simulink model "cartesian_impedance_control"  (R2022b)
settings: Solver=FixedStepDiscrete  StartTime=0.0  StopTime=inf  FixedStep=0.001  RelTol=1e-3
PreLoadFcn:
  | set_param(gcs, 'RTWSystemTargetFile', 'franka_emika_panda.tlc');
  | 
  | demos_common_configs();
  | collision_behavior = ones(1,52)*100;
InitFcn:
  | parameters;
values from neighbouring files (symbols this model uses):
  init_guess_0 = [2.22044604925e-16 2.22044604925e-16 2.22044604925e-16 2.22044604925e-16 2.22044604925e-16 2.22044604925e-16 2.22044604925e-16 2.22044604925e-16 2.22044604925e-16 2.22044604925e-16 2.22044604925e-16 2.22044604925e-16 ... (276 elements, 276x1)]    [mpc_init_guess_test.mat]    (also in parameters.m = param_MPC8_init_guess.init_guess(2,:))
  mpc_init_reference_values = [-0.0348999931742 -2.4612999645 -3.55689998059 2.23979998651 0.0349999704327 -1.24879998892 0 0 0 0 0 0 ... (54 elements, 54x1)]    [mpc_init_ref_test.mat]
  param_weight_init_cell = [100 0 0 0 0 0 0 100 0 0 0 0 ... (180 elements, 1x180)]    [mpc_init_weight_test.mat]
  q_init = [0, -pi/4, 0, -3 * pi/4, 0, pi/2, pi/4]'    [parameters.m]    (also in parameters_franka_fr3.m)
undefined symbols (not defined in the file or in its folder): ctrl_param, param_robot
libraries: franka_simulink_library x5, dspnetwork x2
settings Model: SimulationMode=external  ExtModeTrigDuration=10000  Creator=vasi_ko  LastModifiedBy=rslstudent
settings SolverCC: AlgebraicLoopSolver=TrustRegion
settings DataIOCC: LimitDataPoints=on  SaveFormat=Array  ReturnWorkspaceOutputs=off
settings OptimizationCC: EnhancedBackFolding=on  OptimizeBlockOrder=speed  DifferentSizesBufferReuse=on  OptimizationCustomize=off
settings DebuggingCC: SolverPrmCheckMsg=warning  ParameterTunabilityLossMsg=error  UnconnectedInputMsg=warning  UnconnectedOutputMsg=warning  UnconnectedLineMsg=warning  SFUnexpectedBacktrackingDiag=warning  SFNoUnconditionalDefaultTransitionDiag=warning  SFExecutionAtInitializationDiag=none  SFMachineParentedDataDiag=warning  ArithmeticOperatorsInVariantConditions=warning
settings HardwareCC: ProdBitPerLong=64  ProdHWDeviceType=Intel->x86-64 (Linux 64)
settings ModelReferenceCC: EnableRefExpFcnMdlSchedulingChecks=on  PropagateSignalLabelsOutOfModel=off
settings SFSimCC: SimUseLocalCustomCode=off  MATLABDynamicMemAlloc=off  CustomCodeUndefinedFunction=UseInterfaceOnly  SimTargetLang=C++
settings RTWCC: SystemTargetFile=franka_emika_panda.tlc  RTWUseLocalCustomCode=off  Toolchain=Franka Simulink | gmake (64-bit linux)  BuildConfiguration=Faster Runs  TargetLang=C++
settings CodeAppCC: OperatorAnnotations=on
settings STFCustomTargetCC: TargetLangStandard=C99 (ISO)  ModelReferenceCompliant=off  MatFileLogging=on  GRTInterface=on  UseToolchainInfoCompliant=on  SystemTargetFile=franka_emika_panda.tlc
settings GRTTargetCC: ModelReferenceCompliant=off  ParMdlRefBuildCompliant=off  CompOptLevelCompliant=off  ConcurrentExecutionCompliant=off  CombineOutputUpdateFcns=off  CPPClassGenCompliant=off  GRTInterface=on  ExtModeStaticAlloc=on  ExtModeTransport=1  ExtModeMexFile=ext_xcp  ExtModeIntrfLevel=Level2 - Open
settings ConfigComp: CovMetricSettings=dw  CovSaveCumulativeToWorkspaceVar=on  CovSaveSingleToWorkspaceVar=on  CovExternalEMLEnable=off  CovSFcnEnable=off

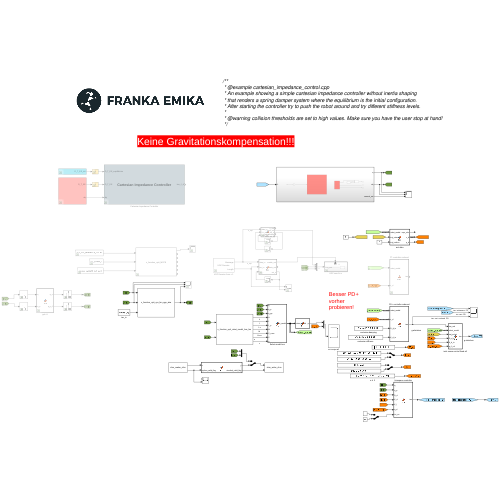
[thumbnail: Simulink's stored preview of the top-level diagram]
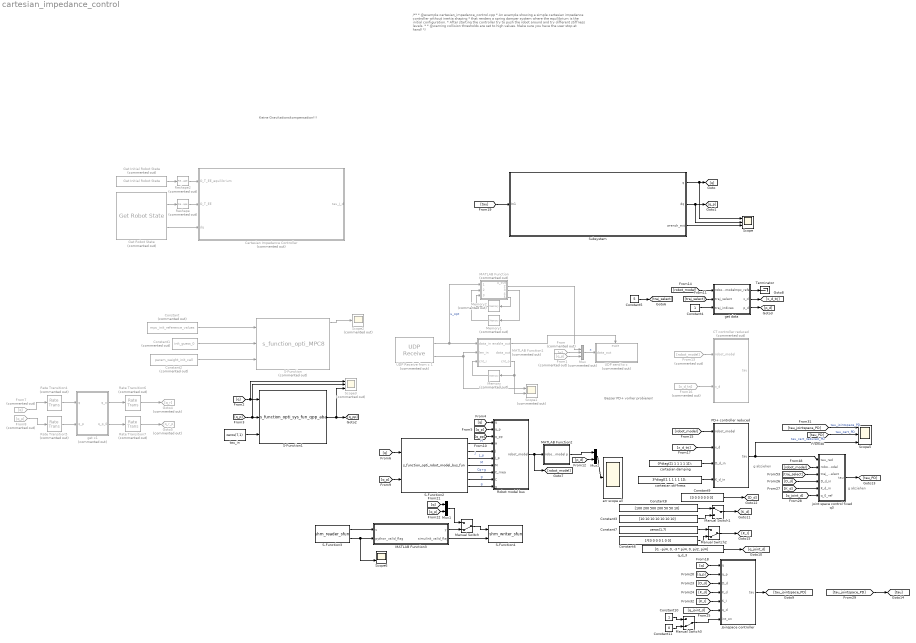
== system cartesian_impedance_control ==
  note: g abziehen
  note: Keine Gravitationskompensation!!!
  note: /**
      |  * @example cartesian_impedance_control.cpp
      |  * An example showing a simple cartesian impedance controller without inertia shaping
      |  * that renders a spring damper system where the equilibrium is the initial configuration.
      |  * After starting the controller try to push the robot around and try different stiffness levels.
      |  *
      |  * @warning collision thresholds are set to high values. Make sure you have the user stop at hand!
      |  */
  note: Besser PD+ vorher probieren!
  note: g abziehen
  CT controller reduced : MATLAB Function  Commented=on  TreatAsAtomicUnit=on
  Cartesian Impedance Controller : Subsystem  Commented=on
      mask Display:
      | disp('{\bf\fontsize{18}Cartesian Impedance Controller}', 'texmode','on');
      | 
      | block_icon('Controller')
      | 
      | port_label('output',1,'tau_J_d');
      | 
      | port_label('input',1,'O_T_EE_equilibrium');
      | port_label('input',2,'O_T_EE');
      | port_label('input',3,'dq');
  Constant : Constant  Commented=on  Value=mpc_init_reference_values
  Constant1 : Constant  Commented=on  Value=init_guess_0
  Constant10 : Constant
  Constant11 : Constant  Value=0
  Constant2 : Constant  Commented=on  Value=param_weight_init_cell
  Constant3 : Constant  Value=[10 10 10 10 10 10 10]
  Constant4 : Constant
  Constant5 : Constant  Value=5
  Constant6 : Constant  Value=1*[0 0 0 0 1 0 0]
  Constant7 : Constant  Value=zeros(1,7)
  Constant8 : Constant  Value=[100 200 500 200 50 50 10]
  Constant9 : Constant  Value=[0 0 0 0 0 0 0]
  From : From  Commented=on  GotoTag=q
  From1 : From  Commented=on  GotoTag=q_p
  From13 : From  Commented=on  GotoTag=robot_model
  From16 : From  Commented=on  GotoTag=x_d_trj
  From7 : From  Commented=on  GotoTag=q
  From8 : From  Commented=on  GotoTag=q_p
  Get Initial Robot State : franka_simulink_library/Get Initial Robot State  Commented=on  robot_ip=robot_ip  signals_requested='O_T_EE'
      settings: SourceProductName=Franka Emika Simulink Support Package
  Get Robot State : franka_simulink_library/Get Robot State  Commented=on  robot_ip=robot_ip  signals_requested='O_T_EE dq'
      settings: SourceProductName=Franka Emika Simulink Support Package
  Goto4 : Goto  Commented=on  GotoTag=q_r
  Goto5 : Goto  Commented=on  GotoTag=q_r_p
  Joinspace controller : MATLAB Function  TreatAsAtomicUnit=on
  MATLAB Function : MATLAB Function  Commented=on  TreatAsAtomicUnit=on
  MATLAB Function1 : MATLAB Function  Commented=on  TreatAsAtomicUnit=on
  MATLAB Function2 : MATLAB Function  TreatAsAtomicUnit=on
  MATLAB Function3 : MATLAB Function  TreatAsAtomicUnit=on
  Manual Switch : ManualSwitch  CurrentSetting=0
  Manual Switch1 : ManualSwitch
  Manual Switch2 : ManualSwitch  CurrentSetting=0
  Manual Switch3 : ManualSwitch  CurrentSetting=0
  Memory : Memory  Commented=on
  Memory1 : Memory  Commented=on
  Memory2 : Memory  Commented=on
  Mux : Mux  Commented=on  Inputs=3
  Mux1 : Mux  Inputs=2
  Mux2 : Mux  Inputs=2
  PD+ controller reduced : MATLAB Function  TreatAsAtomicUnit=on
  Rate Transition4 : RateTransition  Commented=on  OutPortSampleTime=1e-2
  Rate Transition5 : RateTransition  Commented=on  OutPortSampleTime=1e-2
  Rate Transition6 : RateTransition  Commented=on
  Rate Transition7 : RateTransition  Commented=on
  Reshape : Reshape  Commented=on  OutputDimensionality=Customize  OutputDimensions=[4,4]
  Reshape2 : Reshape  Commented=on  OutputDimensionality=Customize  OutputDimensions=[4,4]
  Robot model bus : MATLAB Function  TreatAsAtomicUnit=on
  S-Function : S-Function  Commented=on  FunctionName=s_function_opti_MPC8  SFunctionModules='MPC8'  SFunctionDeploymentMode=off  EnableBusSupport=off
  S-Function1 : S-Function  FunctionName=s_function_opti_sys_fun_qpp_aba  SFunctionModules='sys_fun_qpp_aba'  SFunctionDeploymentMode=off  EnableBusSupport=off
  S-Function2 : S-Function  FunctionName=s_function_opti_robot_model_bus_fun  SFunctionModules='robot_model_bus_fun'  SFunctionDeploymentMode=off  EnableBusSupport=off
  S-Function3 : S-Function  FunctionName=shm_reader_sfun  Parameters='data_from_python', 'data_from_python_valid'  SFunctionDeploymentMode=off  EnableBusSupport=off
  S-Function4 : S-Function  FunctionName=shm_writer_sfun  Parameters='data_from_simulink', 'data_from_simulink_valid'  SFunctionDeploymentMode=off  EnableBusSupport=off
  Scope : Scope  NumInputPorts=3
  Scope1 : Scope  Commented=on  NumInputPorts=2
  Scope2 : Scope  Commented=on
  Scope3 : Scope  Commented=on  NumInputPorts=3
  Scope5 : Scope  NumInputPorts=3
  Scope6 : Scope  NumInputPorts=2
  Subsystem : Subsystem
  Terminator : Terminator
  UDP Receive from c 1 : dspnetwork/UDP Receive  Commented=on  localURL='0.0.0.0'  localPort=8080  remoteURL='127.0.0.1'  remotePort=-1  recvBufferSize=8+6*8*5  dims=1+6*5  signalDatatype=double  isComplex=off  isVarSize=off  showBlockingTime=off  blockingTime=0  sampletime=param_global.Ta  blockPlatform=[]
      settings: LibrarySourceBlock=dspsrcs4/UDP Receive
  UDP send to c : Subsystem  Commented=on
  cartesian damping : Constant  Value=0*diag([1 1 1 1 1 1]);
  cartesian stiffness : Constant  Value=3*diag([1 1 1 1 1 1]);
  err scope all : Scope
  get data : MATLAB Function  TreatAsAtomicUnit=on
  get x1 : MATLAB Function  Commented=on  TreatAsAtomicUnit=on
  joint space control fixed q3 : MATLAB Function  TreatAsAtomicUnit=on
  q_d_3 : Constant  Value=[0, -pi/4, 0, -3 * pi/4, 0, pi/2, pi/4]
  tau_in : Constant  Value=zeros(7,1)
  wires:
  Reshape2/1 -> Cartesian Impedance Controller/1(O_T_EE_equilibrium)
  get data/1(mpc_refs) -> Terminator/1
  From16/1 -> CT controller reduced/2(x_d)
  MATLAB Function/3(init_cnt_o) -> Memory1/1
  MATLAB Function/2(send_cnt) -> Mux/1
  [robot_model] -> get data/1(robot_model)
  MATLAB Function1/3(cnt_o) -> Scope1/2, Memory/1
  Get Initial Robot State/1 -> Reshape2/1
  tau_in/1 -> S-Function1/3
  S-Function2/3 -> Robot model bus/6(J_p)  "J_p"
  [x_d_trj] -> PD+ controller reduced/2(x_d)
  Memory1/1 -> MATLAB Function/2(init_cnt)
  Rate Transition7/1 -> Goto5/1
  [q_p] -> Scope3/2, S-Function1/2
  From/1 -> Mux/2
  Subsystem/1(q) -> Scope/1, [q]
  Constant2/1 -> S-Function/3
  Subsystem/2(dq) -> Scope/2, [q_p]
  [robot_model] -> PD+ controller reduced/1(robot_model)
  S-Function2/6 -> Robot model bus/9(C)  "g"
  [q_pp] -> Robot model bus/3(q_pp)
  [q] -> Scope3/1, S-Function1/1
  UDP Receive from c 1/1 -> MATLAB Function/1(data_in), MATLAB Function1/1(data_in)  "u_opt"
  Constant1/1 -> S-Function/2
  Get Robot State/2 -> Cartesian Impedance Controller/3(dq)
  Rate Transition5/1 -> get x1/2(q_p)
  UDP Receive from c 1/2 -> MATLAB Function1/2(len_in), Scope1/1
  MATLAB Function/5(data_cnt_o) -> Memory2/1
  get x1/1(q_o) -> Rate Transition6/1
  From8/1 -> Rate Transition5/1
  From7/1 -> Rate Transition4/1
  get data/2(x_d) -> [x_d_trj]
  S-Function2/5 -> Robot model bus/8(C_rnea)  "Cq+g"
  S-Function1/1 -> [q_pp], Scope3/3
  Rate Transition6/1 -> Goto4/1
  S-Function2/1 -> Robot model bus/4(H)  "H"
  Reshape/1 -> Cartesian Impedance Controller/2(O_T_EE)
  get x1/2(q_p_0) -> Rate Transition7/1
  MATLAB Function1/1(enable_out) -> UDP send to c/Enable
  Mux/1 -> UDP send to c/1(data_out)  "x"
  S-Function2/2 -> Robot model bus/5(J)  "J"
  Get Robot State/1 -> Reshape/1
  S-Function2/4 -> Robot model bus/7(M)  "M"
  Robot model bus/1(robot_model) -> MATLAB Function2/1(robot_model), [robot_model]
  Subsystem/3(wrench_ext) -> Scope/3
  S-Function/1 -> Scope2/1
  Memory/1 -> MATLAB Function1/3(cnt_i)
  Memory2/1 -> MATLAB Function/3(data_cnt)
  From1/1 -> Mux/3
  Constant/1 -> S-Function/1
  From13/1 -> CT controller reduced/1(robot_model)
  S-Function2/7 -> Robot model bus/10(g)  "g"
  Rate Transition4/1 -> get x1/1(q)
  Constant4/1 -> get data/3(traj_indices)
  cartesian stiffness/1 -> PD+ controller reduced/4(K_d_in)
  cartesian damping/1 -> PD+ controller reduced/3(D_d_in)
  Joinspace controller/1(tau) -> [tau_jointspace_PD]
  [tau] -> Subsystem/1(In1)
  [q] -> Joinspace controller/1(q)
  [q_p] -> Joinspace controller/2(q_p)
  S-Function3/1 -> MATLAB Function3/1(u)
  S-Function3/2 -> Scope6/2, MATLAB Function3/2(python_valid_flag)
  MATLAB Function3/2(simulink_valid_flag) -> S-Function4/2
  [q] -> Mux1/1
  [q_p] -> Mux1/2
  MATLAB Function3/1(y) -> Manual Switch/2
  Manual Switch/1 -> S-Function4/1
  Mux1/1 -> Manual Switch/1
  [q] -> Robot model bus/1(q)
  [q_p] -> Robot model bus/2(q_p)
  [q] -> S-Function2/1
  [q_p] -> S-Function2/2
  get data/3(p_d) -> [p_d]
  [p_d] -> Mux2/2
  MATLAB Function2/1(p) -> Mux2/1
  Mux2/1 -> err scope all/1
  [robot_model] -> joint space control fixed q3/2(robot_model)
  PD+ controller reduced/1(tau) -> Scope5/3, joint space control fixed q3/1(tau_red)  "tau_cart_reduced_PD"
  [traj_select] -> joint space control fixed q3/3(traj_select)
  [traj_select] -> get data/2(traj_select)
  Constant5/1 -> [traj_select]
  [q_joint_d] -> Joinspace controller/6(q_d)
  q_d_3/1 -> [q_joint_d]
  [K_d] -> Joinspace controller/4(K_d)
  [D_d] -> Joinspace controller/3(D_d)
  Constant9/1 -> [D_d]
  [D_d] -> joint space control fixed q3/4(D_d_in)
  [K_d] -> joint space control fixed q3/5(K_d_in)
  [q_joint_d] -> joint space control fixed q3/6(q_0_ref)
  joint space control fixed q3/1(tau) -> [tau_PD]
  [tau_jointspace_PD] -> [tau]
  [tau_PD] -> Scope5/2  "tau_cart_PD"
  [tau_jointspace_PD] -> Scope5/1  "tau_jointspace_PD"
  Constant8/1 -> Manual Switch1/1
  Constant3/1 -> Manual Switch1/2
  Manual Switch1/1 -> [K_d]
  [K_I] -> Joinspace controller/5(K_I)
  Manual Switch2/1 -> [K_I]
  Constant6/1 -> Manual Switch2/2
  Constant7/1 -> Manual Switch2/1
  Constant10/1 -> Manual Switch3/1
  Constant11/1 -> Manual Switch3/2
  Manual Switch3/1 -> Joinspace controller/7(int_on)

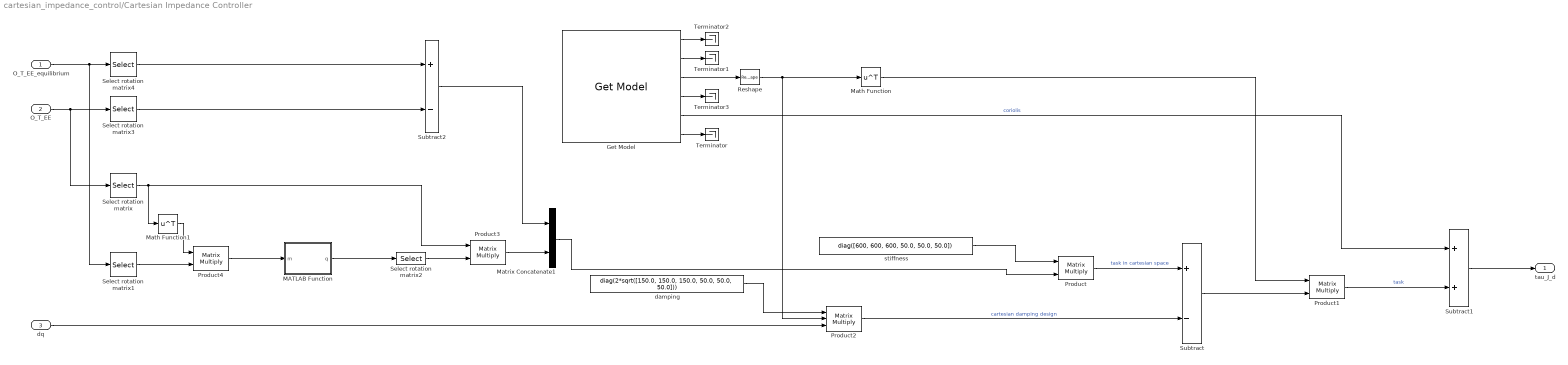
== system cartesian_impedance_control/Cartesian Impedance Controller ==
  O_T_EE_equilibrium : Inport
  O_T_EE : Inport  Port=2
  dq : Inport  Port=3
  Get Model : franka_simulink_library/Get Model  robot_ip=robot_ip
      settings: SourceProductName=Franka Emika Simulink Support Package
  MATLAB Function : MATLAB Function  TreatAsAtomicUnit=on
  Math Function : Math  Operator=transpose  SignedPower=on
  Math Function1 : Math  Operator=transpose  SignedPower=on
  Matrix Concatenate1 : Concatenate
  Product{,1,3..4} (4 alike) : Product  Multiplication=Matrix(*)
  Product2 : Product  Inputs=3  Multiplication=Matrix(*)
  Reshape : Reshape  OutputDimensionality=Customize  OutputDimensions=[6,7]
  Select rotation matrix : Selector  NumberOfDimensions=2  InputPortWidth=3  IndexOptions=Index vector (dialog),Index vector (dialog)  Indices=[1,2,3],[1 2 3]  OutputSizes=1
  Select rotation matrix1 : Selector  NumberOfDimensions=2  InputPortWidth=3  IndexOptions=Index vector (dialog),Index vector (dialog)  Indices=[1,2,3],[1 2 3]  OutputSizes=1
  Select rotation matrix2 : Selector  InputPortWidth=4  IndexOptions=Index vector (dialog)  Indices=[2,3,4]  OutputSizes=1
  Select rotation matrix3 : Selector  NumberOfDimensions=2  InputPortWidth=3  IndexOptions=Index vector (dialog),Index vector (dialog)  Indices=[1,2,3],[4]  OutputSizes=1
  Select rotation matrix4 : Selector  NumberOfDimensions=2  InputPortWidth=3  IndexOptions=Index vector (dialog),Index vector (dialog)  Indices=[1,2,3],[4]  OutputSizes=1
  Subtract : Sum  Inputs=+-
  Subtract1 : Sum
  Subtract2 : Sum  Inputs=+-
  Terminator{,1..3} (4 alike) : Terminator
  damping : Constant  Value=diag(2*sqrt([150.0, 150.0, 150.0, 50.0, 50.0, 50.0]))  VectorParams1D=off
  stiffness : Constant  Value=diag([600, 600, 600, 50.0, 50.0, 50.0])  VectorParams1D=off
  tau_J_d : Outport  VectorParamsAs1DForOutWhenUnconnected=off
  wires:
  Get Model/6 -> Terminator/1
  Get Model/2 -> Terminator1/1
  Get Model/1 -> Terminator2/1
  Get Model/4 -> Terminator3/1
  Get Model/3 -> Reshape/1
  Reshape/1 -> Product2/2, Math Function/1
  stiffness/1 -> Product/1
  Math Function/1 -> Product1/1
  Product/1 -> Subtract/1  "task in cartesian space"
  Product2/1 -> Subtract/2  "cartesian damping design"
  Get Model/5 -> Subtract1/1  "coriolis"
  dq/1 -> Product2/3
  damping/1 -> Product2/1
  Subtract1/1 -> tau_J_d/1
  Product1/1 -> Subtract1/2  "task"
  O_T_EE/1 -> Select rotation matrix3/1, Select rotation matrix/1
  O_T_EE_equilibrium/1 -> Select rotation matrix4/1, Select rotation matrix1/1
  Select rotation matrix4/1 -> Subtract2/1
  Select rotation matrix3/1 -> Subtract2/2
  Subtract2/1 -> Matrix Concatenate1/1
  MATLAB Function/1(q) -> Select rotation matrix2/1
  Product4/1 -> MATLAB Function/1(m)
  Subtract/1 -> Product1/2
  Select rotation matrix2/1 -> Product3/2
  Matrix Concatenate1/1 -> Product/2
  Select rotation matrix/1 -> Math Function1/1, Product3/1
  Product3/1 -> Matrix Concatenate1/2
  Select rotation matrix1/1 -> Product4/2
  Math Function1/1 -> Product4/1

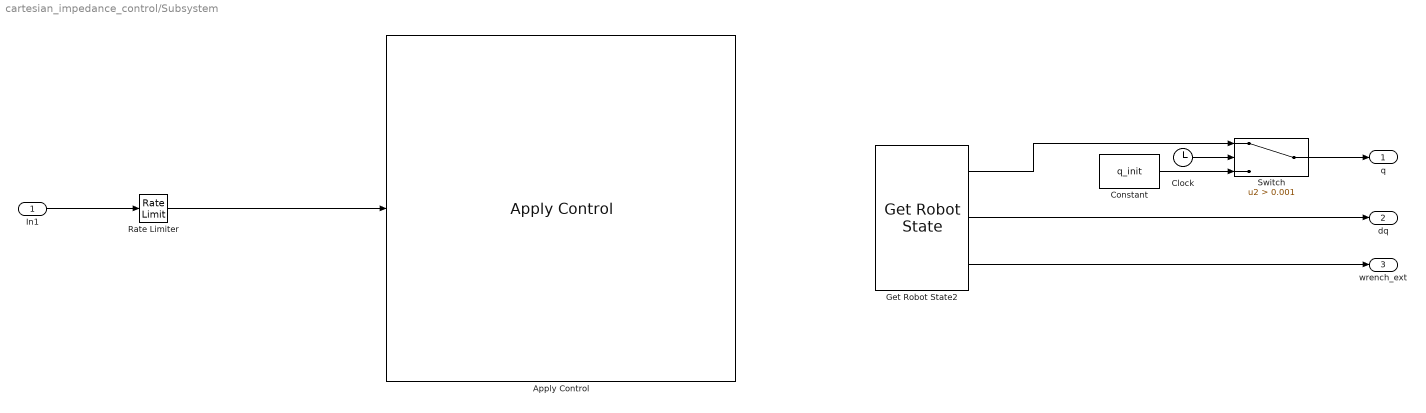
== system cartesian_impedance_control/Subsystem ==
  In1 : Inport
  Apply Control : franka_simulink_library/Apply Control  robot_ip=robot_ip  gripper_attached=off  control_mode=Torque Control  controller_choice=Joint Impedance Controller  elbow_control=on  collision_thresholds=100*ones(1,52)  joint_impedance=joint_impedance  cartesian_impedance=cartesian_impedance  load_inertia=load_inertia  EE_T_K=EE_T_K  init_joint_configuration_req=on  init_joint_configuration=q_init'
      settings: SourceProductName=Franka Emika Simulink Support Package
  Clock : Clock
  Constant : Constant  Value=q_init
  Get Robot State2 : franka_simulink_library/Get Robot State  robot_ip=robot_ip  signals_requested='q dq O_F_ext_hat_K'
      settings: SourceProductName=Franka Emika Simulink Support Package
  Rate Limiter : RateLimiter  RisingSlewLimit=1000  FallingSlewLimit=-1000  SampleTimeMode=inherited
  Switch : Switch  Criteria=u2 > Threshold  Threshold=0.001  SaturateOnIntegerOverflow=off  InputSameDT=off
  q : Outport
  dq : Outport  Port=2
  wrench_ext : Outport  Port=3
  wires:
  Clock/1 -> Switch/2
  Constant/1 -> Switch/3
  Get Robot State2/3 -> wrench_ext/1
  Get Robot State2/2 -> dq/1
  In1/1 -> Rate Limiter/1
  Get Robot State2/1 -> Switch/1
  Switch/1 -> q/1
  Rate Limiter/1 -> Apply Control/1

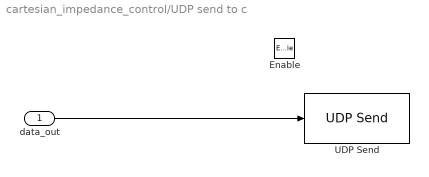
== system cartesian_impedance_control/UDP send to c ==
  data_out : Inport
  Enable : EnablePort
  UDP Send : dspnetwork/UDP Send  remoteURL='127.0.0.1'  remotePort=8081  localURL='0.0.0.0'  localPortSource=Automatically determine  localPort=8081  sendBufferSize=104  sampletime=-1  blockPlatform=[]  separateLengthPort=0
      settings: LibrarySourceBlock=dspsnks4/UDP Send
  wires:
  data_out/1 -> UDP Send/1

== matlab function cartesian_impedance_control/get data ==
  settings: updateMethod=DISCRETE  sampleTime=param_global.Ta
  data: mpc_refs output; robot_model input Bus: robot_model; traj_select input; param_traj_data parameter; traj_indices input; x_d output Bus: x_d; p_d output
function [mpc_refs, x_d, p_d]  = fcn(robot_model, traj_select, param_traj_data, traj_indices)
persistent cnt;

if(isempty(cnt))
    cnt = 1;
end

traj_indices = traj_indices + (cnt-1);

% Parameters
q    = robot_model.q;      % generalized coordinates
q_p  = robot_model.q_p;  % time derivative of generalized coordinates

x_k = [q;q_p];

% Assemble vector of recieved output measurements
p_d     = param_traj_data.p_d(   1:3, traj_indices, traj_select);
q_d     = param_traj_data.q_d(   1:4, traj_indices, traj_select);

y_d = [p_d; q_d];

%% Reference out
mpc_refs = [x_k(:); y_d(:)];

%% Offline Trajectory out
x_d.p_d            = param_traj_data.p_d(           :,    cnt, traj_select);
x_d.p_d_p          = param_traj_data.p_d_p(         :,    cnt, traj_select);
x_d.p_d_pp         = param_traj_data.p_d_pp(        :,    cnt, traj_select);
x_d.Phi_d          = param_traj_data.Phi_d(         :,    cnt, traj_select);
x_d.Phi_d_p        = param_traj_data.Phi_d_p(       :,    cnt, traj_select);
x_d.Phi_d_pp       = param_traj_data.Phi_d_pp(      :,    cnt, traj_select);
x_d.R_d            = param_traj_data.R_d(           :, :, cnt, traj_select);
x_d.q_d            = param_traj_data.q_d(           :,    cnt, traj_select);
x_d.q_d_p          = param_traj_data.q_d_p(         :,    cnt, traj_select);
x_d.q_d_pp         = param_traj_data.q_d_pp(        :,    cnt, traj_select);
x_d.omega_d        = param_traj_data.omega_d(       :,    cnt, traj_select);
x_d.omega_d_p      = param_traj_data.omega_d_p(     :,    cnt, traj_select);
x_d.alpha_d        = param_traj_data.alpha_d(       :,    cnt, traj_select);
x_d.alpha_d_p      = param_traj_data.alpha_d_p(     :,    cnt, traj_select);
x_d.alpha_d_pp     = param_traj_data.alpha_d_pp(    :,    cnt, traj_select);
x_d.rot_ax_d       = param_traj_data.rot_ax_d(      :,    cnt, traj_select);
x_d.alpha_d_offset = param_traj_data.alpha_d_offset(:,    cnt, traj_select);
x_d.q_d_rel        = param_traj_data.q_d_rel(       :,    cnt, traj_select);

%if(cnt < param_traj_data.N)
    %cnt = cnt+1;
%end

== matlab function cartesian_impedance_control/Joinspace controller ==
  settings: updateMethod=DISCRETE  sampleTime=param_global.Ta
  data: tau output; q input; q_p input; D_d input; K_d input; K_I input; q_d input; int_on input
function tau  = fcn(q, q_p, D_d, K_d, K_I, q_d, int_on)

% Parameters
persistent e_I;
if(isempty(e_I))
    e_I = zeros(7,1);
end

e_q = q - q_d;
tau = -diag(D_d)*q_p -diag(K_d)*e_q;

if(int_on == 1)
    e_I = e_I + e_q;
    tau_I = -diag(K_I) * e_I;
else
    e_I = zeros(7,1);
    tau_I = zeros(7,1);
end
tau = tau + tau_I;

== matlab function cartesian_impedance_control/MATLAB Function3 ==
  settings: updateMethod=DISCRETE  sampleTime=1e-3
  data: u input; y output; simulink_valid_flag output; python_valid_flag input
function [y, simulink_valid_flag] = fcn(u, python_valid_flag)

if(python_valid_flag == 1)
    y = u(1:14);
    simulink_valid_flag = 1;
else
    y = zeros(14,1);
    simulink_valid_flag = 0;
end

== matlab function cartesian_impedance_control/CT controller reduced ==
  settings: updateMethod=DISCRETE  sampleTime=param_global.Ta
  data: tau output; robot_model input Bus: robot_model; x_d input Bus: x_d; ctrl_param parameter; param_robot parameter
function tau  = fcn(robot_model, x_d, ctrl_param, param_robot)

% Parameters
%q = robot_model.q;      % generalized coordinates
q_p = robot_model.q_p;  % time derivative of generalized coordinates

M = robot_model.M;      % inertia matrix
%C = robot_model.C;      % coriolis matrix
%g = robot_model.g;      % gravitational forces
%C_rnea = C*q_p + g;
C_rnea = robot_model.C_rnea; % C_rnea(q, q_p) = C(q, q_p)q_p + g(q) = n(q, q_p)

J = robot_model.J;      % geometric jacobian to end-effector
J_p = robot_model.J_p;  % time derivative of geometric jacobian to end-effector

H = robot_model.H;

n = param_robot.n_red;
n_indices = param_robot.n_indices;

yt_indices = param_robot.yt_indices;
yr_indices = param_robot.yr_indices;
y_indices =  [yt_indices 3+yr_indices];

m = numel(yt_indices) + numel(yr_indices);

M_red = M(n_indices, n_indices);
C_rnea_red = C_rnea(n_indices);

J_red = J(y_indices, n_indices);
J_p_red = J_p(y_indices, :);

% Control parameters
Kp1 = ctrl_param.ct.Kp1(y_indices, y_indices);
Kd1 = ctrl_param.ct.Kd1(y_indices, y_indices);

% Current Pose of Endeffector
x_p = J*q_p;

p = H(yt_indices,4);
R = H(1:3,1:3);
p_p  = x_p(yt_indices);
omega_e = x_p(3+yr_indices); % Drehwinkelgeschwindigkeit des Endeffektors

% Desired Trajectory
p_d    = x_d.p_d(yt_indices);
p_d_p  = x_d.p_d_p(yt_indices);
p_d_pp = x_d.p_d_pp(yt_indices);

R_d = x_d.R_d;
omega_d = x_d.omega_d(yr_indices);
omega_d_p = x_d.omega_d_p(yr_indices);

% Errors
RR = R*R_d';
q_err_tmp   = rotm2quat_v4(RR);
q_err = q_err_tmp(1+yr_indices);

x_err   = [p-p_d;      q_err];   % Error as quaternion
x_err_p = [p_p-p_d_p;  omega_e-omega_d];
x_d_pp  = [p_d_pp;     omega_d_p];


% CT control law
%% Cartesian Endeffector Pose

sing_method = ctrl_param.regularization.mode;

if(sing_method == 0)
    v = J_red\(x_d_pp - Kd1*x_err_p - Kp1*x_err - J_p_red*q_p);
elseif(sing_method == 1) % add +k*E
    k = ctrl_param.regularization.k;
    J_pinv = (J_red'*J_red + k*eye(n))\J_red';
    v = J_pinv * (x_d_pp - Kd1*x_err_p - Kp1*x_err - J_p_red*q_p);
elseif(sing_method == 2) % add +lambda*E
    W_bar_N = ctrl_param.regularization.W_bar_N(n_indices);
    W_E = ctrl_param.regularization.W_E(y_indices, y_indices);

    e = x_err;
    E_k = 1/2 * e' * W_E * e;
    W_N = eye(n)*E_k + W_bar_N;

    [~, S, V] = svd(sqrt(W_E)*J_red);

    S_nonzero = diag(diag(S)); % get only nonzero sing values

    H_k = V*(S_nonzero^2)*V' + W_N;
    J_pinv = H_k\J_red';
    v = J_pinv * (x_d_pp - Kd1*x_err_p - Kp1*x_err - J_p_red*q_p);
    %v = H_k \ J_red' * (x_d_pp - Kd1*x_err_p - Kp1*x_err - J_p*q_p);
elseif(sing_method == 3) % remove small singular values
    % Perform SVD
    [U, S, V] = svd(J_red);
    
    % Set a threshold for small singular values
    epsilon = ctrl_param.regularization.eps; % Adjust epsilon as needed
    
    % Threshold small singular values in S
    S_new = diag(max(diag(S), epsilon));  % Creates a diagonal matrix with thresholded values
    S(1:n, 1:n) = S_new;
    
    % Reconstruct the matrix with modified singular values
    J_new = U * S * V';
    J_pinv = pinv(J_new);
    v = J_pinv * (x_d_pp - Kd1*x_err_p - Kp1*x_err - J_p_red*q_p);
elseif(sing_method == 4) % collinearity   
    if(rank(J_red, 1e-1) < m)
        J_tilde = J_red./vecnorm(J_red);
        JJ_colin = J_tilde'*J_tilde;
        [i,j] = find(abs(tril(JJ_colin) - eye(n)) > ctrl_param.regularization.eps_collinear);

        J_red(:, j) = 0;
        
        J_pinv = pinv(J_red);
        
        v = J_pinv * (x_d_pp - Kd1*x_err_p - Kp1*x_err - J_p_red*q_p);% - D_n * q_p_nullspace - K_n * (q_nullspace - q_d_nullspace);
        v(j) = 0;
    else
        v = J_red \ (x_d_pp - Kd1*x_err_p - Kp1*x_err - J_p_red*q_p);% - D_n * q_p_nullspace - K_n * (q_nullspace - q_d_nullspace);
    end
else%if(sing_method == 5) % nach Steinboeck Optreg
    J_scale = 1./vecnorm(J_red);
    J_tilde = J_red.*J_scale;
    JJ_colin = J_tilde'*J_tilde;
    %[V, D] = eig(JJ_colin);

    [U, D, V] = svd(JJ_colin);

    V_new = real(V(:, real(diag(D)) > ctrl_param.regularization.lambda_min));

    T_bar = J_scale' .* V_new;

    J_new = J_red*T_bar;

    v = T_bar * ( J_new \ (x_d_pp - Kd1*x_err_p - Kp1*x_err - J_p_red*q_p) );
end

tau = M_red*v + C_rnea_red;
%if(max(abs(tau)) > 200)
%    disp('no');
%end

== matlab function cartesian_impedance_control/PD+ controller reduced ==
  settings: updateMethod=DISCRETE  sampleTime=param_global.Ta
  data: tau output; robot_model input Bus: robot_model; x_d input Bus: x_d; D_d_in input; K_d_in input; ctrl_param parameter; param_robot parameter
function tau  = fcn(robot_model, x_d, D_d_in, K_d_in, ctrl_param, param_robot)

% Parameters
%q = robot_model.q;      % generalized coordinates
q_p = robot_model.q_p;  % time derivative of generalized coordinates

M = robot_model.M;      % inertia matrix
C = robot_model.C;      % coriolis matrix
%g = robot_model.g;      % gravitational forces
%C_rnea = robot_model.C_rnea; % C_rnea(q, q_p) = C(q, q_p)q_p + g(q) = n(q, q_p)

J = robot_model.J;      % geometric jacobian to end-effector

J_p = robot_model.J_p;  % time derivative of geometric jacobian to end-effector
H = robot_model.H;

n = param_robot.n_red;
n_indices = param_robot.n_indices;

yt_indices = param_robot.yt_indices;
yr_indices = param_robot.yr_indices;
y_indices =  [yt_indices 3+yr_indices];

m = numel(yt_indices) + numel(yr_indices);

M_red = M(n_indices, n_indices);
C_red = C(n_indices, n_indices);
%C_rnea_red = C_rnea(n_indices);

J_red = J(y_indices, n_indices);
J_p_red = J_p(y_indices, n_indices);

%g_red = g(n_indices);

% Control parameters
%D_d = ctrl_param.pd.D_d(y_indices, y_indices);
%K_d = ctrl_param.pd.K_d(y_indices, y_indices);

D_d = D_d_in(y_indices, y_indices);
K_d = K_d_in(y_indices, y_indices);

% Current Pose of Endeffector
x_p = J*q_p;

p = H(yt_indices,4);
R = H(1:3,1:3);
p_p  = x_p(yt_indices);
omega_e = x_p(3+yr_indices); % Drehwinkelgeschwindigkeit des Endeffektors

% Desired Trajectory
p_d    = x_d.p_d(yt_indices);
p_d_p  = x_d.p_d_p(yt_indices);
p_d_pp = x_d.p_d_pp(yt_indices);

R_d = x_d.R_d;
omega_d = x_d.omega_d(yr_indices);
omega_d_p = x_d.omega_d_p(yr_indices);

% Errors
RR = R*R_d';
q_err_tmp   = rotm2quat_v4(RR);
q_err = q_err_tmp(1+yr_indices);

x_err   = [p-p_d;      q_err];   % Error as quaternion
x_err_p = [p_p-p_d_p;  omega_e-omega_d];
x_d_p   = [p_d_p;      omega_d];
x_d_pp  = [p_d_pp;     omega_d_p];


% CT control law
%% Cartesian Endeffector Pose

sing_method = ctrl_param.regularization.mode;
j = [];

if(sing_method == 0)
    J_pinv = J_red\eye(m);
elseif(sing_method == 1) % add +k*E
    k = ctrl_param.regularization.k;
    J_pinv = (J_red'*J_red + k*eye(n))\J_red';
elseif(sing_method == 2) % add +lambda*E
    W_bar_N = ctrl_param.regularization.W_bar_N(n_indices);
    W_E = ctrl_param.regularization.W_E(y_indices, y_indices);

    e = x_err;
    E_k = 1/2 * e' * W_E * e;
    W_N = eye(n)*E_k + W_bar_N;

    [~, S, V] = svd(sqrt(W_E)*J_red);

    S_nonzero = diag(diag(S)); % get only nonzero sing values

    H_k = V*(S_nonzero^2)*V' + W_N;
    J_pinv = H_k\J_red';
elseif(sing_method == 3) % remove small singular values
    % Perform SVD
    [U, S, V] = svd(J_red);
    
    % Set a threshold for small singular values
    epsilon = ctrl_param.regularization.eps; % Adjust epsilon as needed
    
    % Threshold small singular values in S
    S_new = diag(max(diag(S), epsilon));  % Creates a diagonal matrix with thresholded values
    S(1:n, 1:n) = S_new;
    
    % Reconstruct the matrix with modified singular values
    J_new = U * S * V';
    J_pinv = pinv(J_new);
elseif(sing_method == 4) % collinearity   
    if(rank(J_red, 1e-1) < m)
        J_tilde = J_red./vecnorm(J_red);
        JJ_colin = J_tilde'*J_tilde;
        [i,j] = find(abs(tril(JJ_colin) - eye(n)) > ctrl_param.regularization.eps_collinear);

        J_red(:, j) = 0;
        
        J_pinv = pinv(J_red);
    else
        J_pinv = J_red\eye(m);
    end
else%if(sing_method == 5) % nach Steinboeck Optreg
    J_scale = 1./vecnorm(J_red);
    J_tilde = J_red.*J_scale;
    JJ_colin = J_tilde'*J_tilde;
    %[V, D] = eig(JJ_colin);

    [U, D, V] = svd(JJ_colin);

    V_new = real(V(:, real(diag(D)) > ctrl_param.regularization.lambda_min));

    T_bar = J_scale' .* V_new;

    J_new = J_red*T_bar;

    J_pinv = T_bar * (J_new \ eye(m));
end

J_pinv_T = J_pinv';
Lambda = J_pinv_T*M_red*J_pinv;
Lambda = 1/2 * (Lambda + Lambda');
mu = J_pinv_T*(C_red - M_red*J_pinv*J_p_red)*J_pinv;
%mu = Lambda * (J / (M) * C - J_p);

%F_g = J_pinv_T*g_red; % IGNORED

%Lambda = inv(J)' * (C - M * inv(J)*J_p)*inv(J);
%mu = inv(J)' * (C - M*inv(J)*J_p)*inv(J);
%F_g = inv(J)'*g;

F_red = Lambda*x_d_pp + mu*x_d_p - D_d*x_err_p - K_d*x_err; % F_g is ignored

tau = J_red' * F_red;

%tau = g + J'* (-K_d * x_err - D_d * x_err_p);

%if(sing_method == 4)
%    tau(j) = 0;
%end

%if(max(abs(tau)) > 200)
%    disp('no');
%end

== matlab function cartesian_impedance_control/joint space control fixed q3 ==
  data: tau_red input size=param_robot.n_red; tau output; robot_model input Bus: robot_model; traj_select input; param_robot parameter; D_d_in input; K_d_in input; q_0_ref input; ctrl_param parameter
function tau = fcn(tau_red, robot_model, traj_select, param_robot, D_d_in, K_d_in, q_0_ref, ctrl_param)

%g = robot_model.g;
q = robot_model.q;
q_p = robot_model.q_p;

n_indices = param_robot.n_indices;
n_indices_fixed = param_robot.n_indices_fixed;

%q_0_ref_fixed = param_traj.q_0(n_indices_fixed, traj_select);

n_DOF = param_robot.n_DOF;

q_0_ref_fix = q_0_ref(n_indices_fixed);
q_fix = q(n_indices_fixed);
q_p_fix = q_p(n_indices_fixed);
%g_fix = g(n_indices_fixed);

%D_d = ctrl_param.pd.D_d_jointspace(n_indices_fixed, n_indices_fixed);
%K_d = ctrl_param.pd.K_d_jointspace(n_indices_fixed, n_indices_fixed);
D_d = diag(D_d_in(n_indices_fixed));
K_d = diag(K_d_in(n_indices_fixed));

tau_fix_q = -K_d * (q_fix - q_0_ref_fix) -D_d*q_p_fix;%g_fix = 0;
%tau_fix_q = g_fix;

tau_tmp = zeros(n_DOF, 1);
tau_tmp(n_indices) = tau_red;
tau_tmp(n_indices_fixed) = tau_fix_q;

tau = tau_tmp;

== matlab function cartesian_impedance_control/Robot model bus ==
  settings: updateMethod=DISCRETE  sampleTime=param_global.Ta
  data: q input; q_p input; q_pp input; H input; J input; J_p input; M input; C_rnea input; C input; g input; robot_model output Bus: robot_model
function robot_model = fcn(q, q_p, q_pp, H, J, J_p, M, C_rnea, C, g)
% Parameters
robot_model=struct();
robot_model.q=q;                    % generalized coordinates
robot_model.q_p=q_p;                % time derivative of generalized coordinates
robot_model.q_pp=q_pp;
robot_model.H=H;
robot_model.J=J;
robot_model.J_p=J_p;
robot_model.M=M;
robot_model.C_rnea=C_rnea; % C_rnea(q, q_p) = C(q, q_p)q_p + g(q) = n(q, q_p)
robot_model.C=C; % C_rnea(q, q_p) = C(q, q_p)q_p + g(q) = n(q, q_p)
robot_model.g=g;
end

== matlab function cartesian_impedance_control/MATLAB Function1 ==
  settings: updateMethod=DISCRETE  sampleTime=param_global.Ta
  data: enable_out output; data_in input; len_in input; data_out output; cnt_i input; cnt_o output
function [enable_out, data_out, cnt_o] = fcn(data_in, len_in, cnt_i)

if(len_in > 0)
    cnt_o = cnt_i + 1;
else
    cnt_o = cnt_i;
end

enable_out = 1;
data_out = [-0.0349; -2.4613; -3.5569; 2.2398; 0.0350; -1.2488; 1; 2; 3; 4; 5; 6];

== matlab function cartesian_impedance_control/Cartesian Impedance Controller/MATLAB Function ==
  data: m input; q output
function q = rotm2quat(m)

m00 = m(1,1);
m01 = m(1,2);
m02 = m(1,3);

m10 = m(2,1);
m11 = m(2,2);
m12 = m(2,3);

m20 = m(3,1);
m21 = m(3,2);
m22 = m(3,3);

tr = m00 + m11 + m22;

if (tr > 0) 
  S = sqrt(tr+1.0) * 2; % S=4*qw 
  qw = 0.25 * S;
  qx = (m21 - m12) / S;
  qy = (m02 - m20) / S; 
  qz = (m10 - m01) / S; 
elseif ((m00 > m11) && (m00 > m22))
  S = sqrt(1.0 + m00 - m11 - m22) * 2;  %S=4*qx 
  qw = (m21 - m12) / S;
  qx = 0.25 * S;
  qy = (m01 + m10) / S; 
  qz = (m02 + m20) / S; 
elseif (m11 > m22) 
  S = sqrt(1.0 + m11 - m00 - m22) * 2; % S=4*qy
  qw = (m02 - m20) / S;
  qx = (m01 + m10) / S; 
  qy = 0.25 * S;
  qz = (m12 + m21) / S; 
else 
  S = sqrt(1.0 + m22 - m00 - m11) * 2; % S=4*qz
  qw = (m10 - m01) / S;
  qx = (m02 + m20) / S;
  qy = (m12 + m21) / S;
  qz = 0.25 * S;
end

q = [qw,qx,qy,qz]';

== matlab function cartesian_impedance_control/get x1 ==
  data: q input; q_o output; q_p input; q_p_0 output
function [q_o, q_p_0] = fcn(q, q_p)

q_o = [q(1:2); q(4:7)];
q_p_0 = [q_p(1:2); q_p(4:7)];

== matlab function cartesian_impedance_control/MATLAB Function2 ==
  data: p output; robot_model input Bus: robot_model
function p  = fcn(robot_model)

H = robot_model.H;
p = H(1:3, 4);

== matlab function cartesian_impedance_control/MATLAB Function ==
  data: data_in input; u_out output; send_cnt output; init_cnt_o output; init_cnt input; start_sending output; data_cnt input; data_cnt_o output
function [u_out, send_cnt, init_cnt_o, start_sending, data_cnt_o] = fcn(data_in, init_cnt, data_cnt)



send_cnt = data_in(1);

if(send_cnt == init_cnt)
    data_cnt_o = 1;
    start_sending = 1;
    
    init_cnt_o = init_cnt + 1;
    u_out = data_in(2:7);
else
    if(data_cnt > 4)
        data_cnt_o = 4;
    else
        data_cnt_o = data_cnt + 1;
    end
    disp('data_cnt');
    disp(data_cnt_o);
    u_out = data_in(1+(1:6)*data_cnt_o);
    start_sending = 0;
    init_cnt_o = init_cnt;
end
